simulink model "gm_sampleModel1869_3_sub_sub_sub"  (R2023a)
settings: Solver=VariableStepAuto  StartTime=0.0  StopTime=10.0  RelTol=1e-3
libraries: hdlsllib x3, simulink x3
settings Model: Creator=user1  LastModifiedBy=user1
settings OptimizationCC: BlockReduction=off  ConditionallyExecuteInputs=off
settings DebuggingCC: InheritedTsInSrcMsg=none

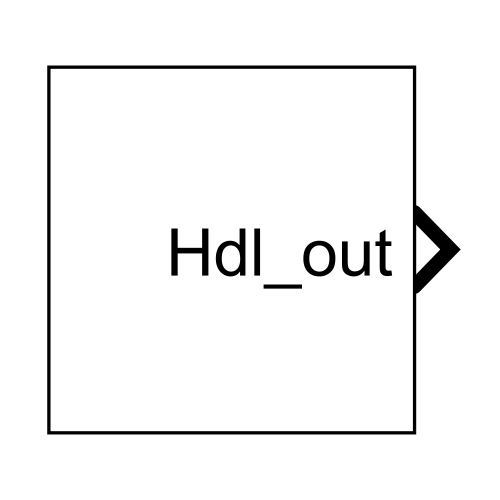
[thumbnail: Simulink's stored preview of the top-level diagram]
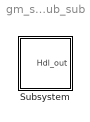
== system gm_sampleModel1869_3_sub_sub_sub ==
  Subsystem : Subsystem

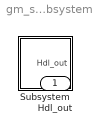
== system gm_sampleModel1869_3_sub_sub_sub/Subsystem ==
  Subsystem : Subsystem
  Hdl_out : Outport  OutDataTypeStr=uint8

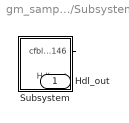
== system gm_sampleModel1869_3_sub_sub_sub/Subsystem/Subsystem ==
  Subsystem : Subsystem
  Hdl_out : Outport  OutDataTypeStr=uint8
  wires:
  Subsystem/1(cfblk146) -> Hdl_out/1

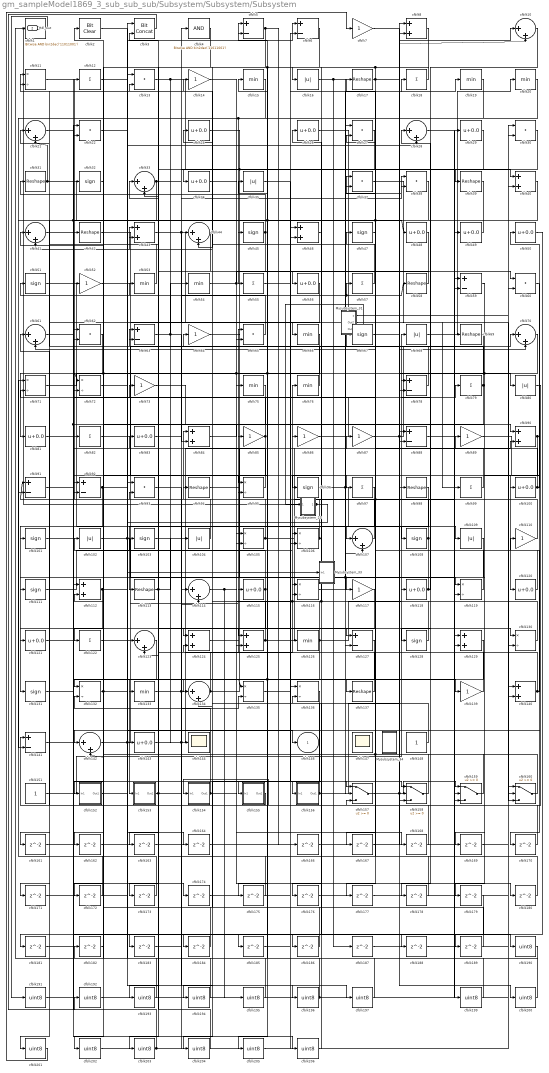
== system gm_sampleModel1869_3_sub_sub_sub/Subsystem/Subsystem/Subsystem ==
  Mysubsystem_23 : Subsystem  TreatAsAtomicUnit=on  RTWFcnName=Mysubsystem_23
      settings: RTWFcnNameOpts=User specified  RTWFileNameOpts=Use function name
  Mysubsystem_31 : Subsystem  TreatAsAtomicUnit=on  RTWFcnName=Mysubsystem_31
      settings: RTWFcnNameOpts=User specified  RTWFileNameOpts=Use function name
  Mysubsystem_33 : Subsystem  TreatAsAtomicUnit=on  RTWFcnName=Mysubsystem_33
      settings: RTWFcnNameOpts=User specified  RTWFileNameOpts=Use function name
  Mysubsystem_34 : Subsystem  TreatAsAtomicUnit=on  RTWFcnName=Mysubsystem_34
      settings: RTWFcnNameOpts=User specified  RTWFileNameOpts=Use function name
  cfblk1 : simulink/Logic and Bit Operations/Bitwise Operator  logicop=AND  UseBitMask=on  BitMask=bin2dec('11011001')  BitMaskRealWorld=Stored Integer
      settings: LibrarySourceBlock=|
      | hdlsllib/Logic and Bit
      | Operations/Bitwise
      | Operator
  cfblk{10,21,28,33,41,44,61,70,107,114,123,134,142} (13 alike) : Sum  Inputs=|++  OutDataTypeStr=uint8
  cfblk{24,26,29,34,48..50,56,81,83,100,115,118,120..121,143} (16 alike) : Bias  Bias=0.0  SaturateOnIntegerOverflow=off
  cfblk{32,45,47,51,67,96,101,103,108,111,128,131} (12 alike) : Signum
  cfblk{16,35,68,80,102,104,109} (7 alike) : Abs  OutDataTypeStr=uint8  SaturateOnIntegerOverflow=off
  cfblk{11,71..72,95,105..106,116,119,130,132,135..136} (12 alike) : Product  Inputs=*/  OutDataTypeStr=uint8  RndMeth=Zero  SaturateOnIntegerOverflow=on
  cfblk{7,14,52,64,73,85..87,89,110,117,139} (12 alike) : Gain  OutDataTypeStr=uint8
  cfblk{8,40,43,46,84,90,112,124..125,129,140} (11 alike) : Sum  OutDataTypeStr=uint8
  cfblk{17,31,39,42,58,69,94,98,113,137} (10 alike) : Reshape
  cfblk{12,18,55,57,79,82,97,99,122} (9 alike) : Sum  Inputs=+  OutDataTypeStr=uint8
  cfblk{15,19..20,53..54,66,75..76,126,133} (10 alike) : MinMax  OutDataTypeStr=uint8
  cfblk{5..6,59,63,78,88,91..92,127,141} (10 alike) : Sum  Inputs=+-  OutDataTypeStr=uint8
  cfblk{13,22,27,30,37..38,60,62,65,93} (10 alike) : DotProduct  OutDataTypeStr=uint8
  cfblk144 : Scope
  cfblk147 : Scope
      settings: Floating=on
  cfblk148 : Constant  OutDataTypeStr=uint8  SampleTime=-1
  cfblk151 : Constant  OutDataTypeStr=uint8  SampleTime=-1
  cfblk152 : Subsystem
      settings: LibrarySourceBlock=|
      | hdlsllib/Ports &
      | Subsystems/Subsystem
  cfblk153 : Subsystem
      settings: LibrarySourceBlock=|
      | hdlsllib/Ports &
      | Subsystems/Subsystem
  cfblk154 : Subsystem
      settings: LibrarySourceBlock=|
      | hdlsllib/Ports &
      | Subsystems/Subsystem
  cfblk155 : Subsystem
      settings: LibrarySourceBlock=|
      | hdlsllib/Ports &
      | Subsystems/Subsystem
  cfblk156 : Subsystem
      settings: LibrarySourceBlock=|
      | hdlsllib/Ports &
      | Subsystems/Subsystem
  cfblk{157..160} (4 alike) : Switch  OutDataTypeStr=uint8  SaturateOnIntegerOverflow=off  InputSameDT=off
  cfblk{161..164,166..189} (28 alike) : Delay  SampleTime=1
  cfblk{190..197,199..206} (16 alike) : DataTypeConversion  OutDataTypeStr=uint8  SaturateOnIntegerOverflow=off  RndMeth=Floor
  cfblk2 : simulink/Logic and Bit Operations/Bit Clear  iBit=0
      settings: LibrarySourceBlock=|
      | hdlsllib/Logic and Bit
      | Operations/Bit Clear
  cfblk3 : hdlsllib/Logic and Bit Operations/Bit Concat  numInputs=2
  cfblk4 : simulink/Logic and Bit Operations/Bitwise Operator  logicop=AND  UseBitMask=on  BitMask=bin2dec('11011001')  BitMaskRealWorld=Stored Integer
      settings: LibrarySourceBlock=|
      | hdlsllib/Logic and Bit
      | Operations/Bitwise
      | Operator
  cfblk146 : Outport  OutDataTypeStr=uint8  VectorParamsAs1DForOutWhenUnconnected=off
  Hdl_out : Outport  Port=2  OutDataTypeStr=uint8
  wires:
  Mysubsystem_31/3(Out3) -> Mysubsystem_23/1(In1)
  Mysubsystem_31/2(Out2) -> cfblk99/1
  Mysubsystem_31/1(y) -> cfblk40/2
  Mysubsystem_23/1(Out1) -> cfblk93/1, Hdl_out/1
  cfblk206/1 -> cfblk136/2
  cfblk141/1 -> cfblk206/1
  cfblk205/1 -> cfblk136/1
  cfblk129/1 -> cfblk205/1
  cfblk204/1 -> cfblk83/1
  cfblk136/1 -> cfblk204/1
  cfblk203/1 -> cfblk60/2, cfblk112/1
  cfblk202/1 -> cfblk4/1
  cfblk75/1 -> cfblk202/1
  cfblk201/1 -> cfblk7/1
  cfblk200/1 -> cfblk62/1
  cfblk7/1 -> cfblk200/1
  cfblk199/1 -> cfblk93/2
  cfblk88/1 -> cfblk199/1
  cfblk197/1 -> cfblk182/1
  cfblk93/1 -> cfblk197/1
  cfblk196/1 -> cfblk95/2, cfblk30/1
  cfblk195/1 -> cfblk2/1
  cfblk194/1 -> cfblk3/2
  cfblk179/1 -> cfblk194/1
  cfblk193/1 -> cfblk3/1
  cfblk27/1 -> cfblk193/1
  cfblk192/1 -> cfblk114/2
  cfblk3/1 -> cfblk192/1
  cfblk191/1 -> cfblk49/1
  cfblk1/1 -> cfblk191/1
  cfblk190/1 -> cfblk1/1
  cfblk161/1 -> cfblk190/1
  cfblk189/1 -> cfblk123/2
  cfblk188/1 -> cfblk159/3
  cfblk187/1 -> cfblk140/1
  cfblk186/1 -> cfblk124/2
  cfblk185/1 -> cfblk6/2
  cfblk184/1 -> cfblk112/2
  cfblk183/1 -> cfblk44/1
  cfblk48/1 -> cfblk183/1
  cfblk182/1 -> cfblk62/2
  cfblk181/1 -> cfblk22/1
  cfblk50/1 -> cfblk181/1
  cfblk180/1 -> cfblk27/2
  cfblk178/1 -> cfblk33/1
  cfblk10/1 -> cfblk178/1
  cfblk177/1 -> cfblk160/1
  cfblk29/1 -> cfblk177/1
  cfblk176/1 -> cfblk160/2
  cfblk97/1 -> cfblk176/1
  cfblk175/1 -> cfblk134/2
  cfblk174/1 -> cfblk46/2
  cfblk101/1 -> cfblk174/1
  cfblk173/1 -> cfblk71/1
  cfblk172/1 -> cfblk92/1
  cfblk32/1 -> cfblk172/1
  cfblk171/1 -> cfblk13/1
  cfblk56/1 -> cfblk171/1
  cfblk170/1 -> cfblk157/3
  cfblk169/1 -> cfblk30/2
  cfblk168/1 -> cfblk61/1
  cfblk167/1 -> cfblk59/2
  cfblk166/1 -> cfblk159/2
  cfblk164/1 -> cfblk8/1
  cfblk72/1 -> cfblk164/1
  cfblk163/1 -> cfblk114/1
  cfblk162/1 -> cfblk119/2
  cfblk61/1 -> cfblk124/1
  cfblk19/1 -> cfblk141/2
  cfblk76/1 -> cfblk11/1
  cfblk112/1 -> cfblk121/1, cfblk28/2
  cfblk65/1 -> cfblk51/1
  cfblk52/1 -> cfblk160/3
  cfblk6/1 -> cfblk44/2, cfblk95/1
  cfblk117/1 -> cfblk155/1(In1)
  cfblk44/1 -> cfblk143/1
  cfblk55/1 -> cfblk19/1
  cfblk102/1 -> cfblk123/1, cfblk129/2
  cfblk14/1 -> cfblk65/2
  cfblk79/1 -> cfblk5/1, cfblk162/1
  cfblk71/1 -> cfblk80/1
  cfblk66/1 -> cfblk135/1, cfblk175/1, cfblk101/1, cfblk125/2
  cfblk28/1 -> cfblk129/1
  cfblk64/1 -> cfblk70/1
  cfblk83/1 -> cfblk58/1, cfblk57/1
  cfblk81/1 -> cfblk134/1
  cfblk58/1 -> cfblk56/1
  cfblk20/1 -> cfblk33/2
  cfblk41/1 -> cfblk97/1
  cfblk133/1 -> cfblk126/1, cfblk38/2
  cfblk57/1 -> cfblk32/1
  cfblk69/1 -> cfblk128/1
  cfblk70/1 -> cfblk78/2, cfblk179/1
  cfblk11/1 -> cfblk48/1, cfblk130/2
  cfblk60/1 -> cfblk100/1
  cfblk49/1 -> cfblk45/1
  cfblk43/1 -> cfblk158/2, cfblk66/1
  cfblk5/1 -> cfblk142/2, cfblk72/1, cfblk166/1
  cfblk94/1 -> cfblk90/2
  cfblk22/1 -> cfblk106/2
  cfblk91/1 -> cfblk79/1
  cfblk63/1 -> cfblk84/2, cfblk54/1
  cfblk4/1 -> cfblk203/1
  cfblk35/1 -> cfblk158/1
  cfblk31/1 -> cfblk105/1, cfblk21/2
  cfblk159/1 -> cfblk37/2, cfblk41/1
  cfblk100/1 -> cfblk50/1, cfblk28/1
  cfblk135/1 -> cfblk87/1
  cfblk38/1 -> cfblk122/1
  cfblk53/1 -> cfblk21/1
  cfblk109/1 -> cfblk133/1
  cfblk111/1 -> cfblk106/1
  cfblk92/1 -> cfblk131/1, cfblk184/1
  cfblk153/1(Out1) -> cfblk73/1, cfblk189/1
  cfblk67/1 -> cfblk8/2
  cfblk78/1 -> cfblk43/1
  cfblk21/1 -> cfblk157/1, cfblk88/2
  cfblk39/1 -> cfblk91/2, cfblk167/1
  cfblk99/1 -> cfblk37/1
  cfblk115/1 -> cfblk72/2, cfblk163/1
  cfblk17/1 -> cfblk107/1, cfblk70/2
  cfblk131/1 -> cfblk22/2
  cfblk80/1 -> cfblk154/1(In1)
  cfblk86/1 -> cfblk59/1
  cfblk118/1 -> cfblk78/1, cfblk111/1
  cfblk96/1 -> cfblk108/1, cfblk158/3, cfblk38/1
  cfblk158/1 -> cfblk15/1
  cfblk73/1 -> cfblk127/2
  cfblk116/1 -> cfblk18/1
  cfblk152/1(Out1) -> cfblk6/1
  cfblk137/1 -> cfblk14/1
  cfblk142/1 -> Mysubsystem_33/1(In1), cfblk115/1
  cfblk59/1 -> cfblk119/1
  cfblk12/1 -> cfblk139/1
  cfblk113/1 -> cfblk13/2, cfblk104/1
  cfblk13/1 -> cfblk40/1, cfblk144/1
  cfblk123/1 -> cfblk153/1(In1)
  cfblk84/1 -> cfblk90/1
  cfblk108/1 -> cfblk157/2, cfblk161/1, cfblk5/2
  cfblk120/1 -> cfblk91/1, cfblk71/2
  cfblk37/1 -> cfblk140/2
  cfblk18/1 -> cfblk16/1
  cfblk85/1 -> cfblk132/1, cfblk53/1
  cfblk104/1 -> cfblk63/1
  cfblk105/1 -> cfblk69/1, cfblk24/1
  cfblk90/1 -> cfblk169/1, cfblk170/1
  cfblk42/1 -> cfblk120/1
  cfblk132/1 -> cfblk52/1, cfblk146/1
  cfblk121/1 -> cfblk82/1
  cfblk134/1 -> cfblk46/1, cfblk103/1
  cfblk47/1 -> cfblk17/1
  cfblk16/1 -> cfblk130/1, cfblk187/1
  cfblk119/1 -> cfblk61/2
  cfblk54/1 -> cfblk60/1, cfblk180/1
  cfblk46/1 -> cfblk96/1
  cfblk154/1(Out1) -> cfblk132/2, cfblk168/1
  cfblk160/1 -> cfblk47/1, cfblk63/2
  cfblk106/1 -> cfblk42/1, cfblk156/1(In1)
  cfblk148/1 -> cfblk102/1
  cfblk127/1 -> cfblk152/1(In1)
  cfblk130/1 -> cfblk35/1
  cfblk34/1 -> cfblk75/1
  cfblk157/1 -> cfblk159/1, cfblk10/1
  cfblk124/1 -> cfblk127/1
  cfblk156/1(Out1) -> cfblk88/1, cfblk11/2
  cfblk2/1 -> cfblk196/1
  cfblk15/1 -> cfblk55/1, cfblk173/1
  cfblk45/1 -> cfblk31/1, cfblk105/2
  cfblk26/1 -> cfblk98/1
  cfblk125/1 -> cfblk89/1, cfblk41/2
  cfblk95/1 -> cfblk12/1
  cfblk62/1 -> cfblk81/1
  cfblk87/1 -> cfblk29/1, cfblk10/2
  cfblk51/1 -> cfblk109/1
  cfblk33/1 -> cfblk39/1, cfblk92/2
  cfblk98/1 -> cfblk113/1
  cfblk122/1 -> cfblk64/1
  cfblk128/1 -> cfblk94/1, cfblk116/1, cfblk26/1
  cfblk40/1 -> cfblk125/1, cfblk201/1
  cfblk143/1 -> cfblk27/1, cfblk135/2, cfblk188/1
  cfblk155/1(Out1) -> cfblk141/1
  cfblk151/1 -> cfblk118/1
  cfblk126/1 -> cfblk68/1, cfblk43/2, cfblk185/1
  cfblk103/1 -> cfblk85/1
  cfblk107/1 -> cfblk84/1
  cfblk139/1 -> cfblk65/1
  cfblk24/1 -> cfblk117/1, cfblk107/2
  cfblk89/1 -> cfblk142/1
  cfblk8/1 -> cfblk137/1, cfblk186/1
  cfblk30/1 -> cfblk34/1
  cfblk140/1 -> cfblk86/1, cfblk110/1
  cfblk114/1 -> cfblk116/2, cfblk195/1
  cfblk68/1 -> cfblk20/1
  cfblk82/1 -> cfblk67/1
  cfblk110/1 -> cfblk76/1

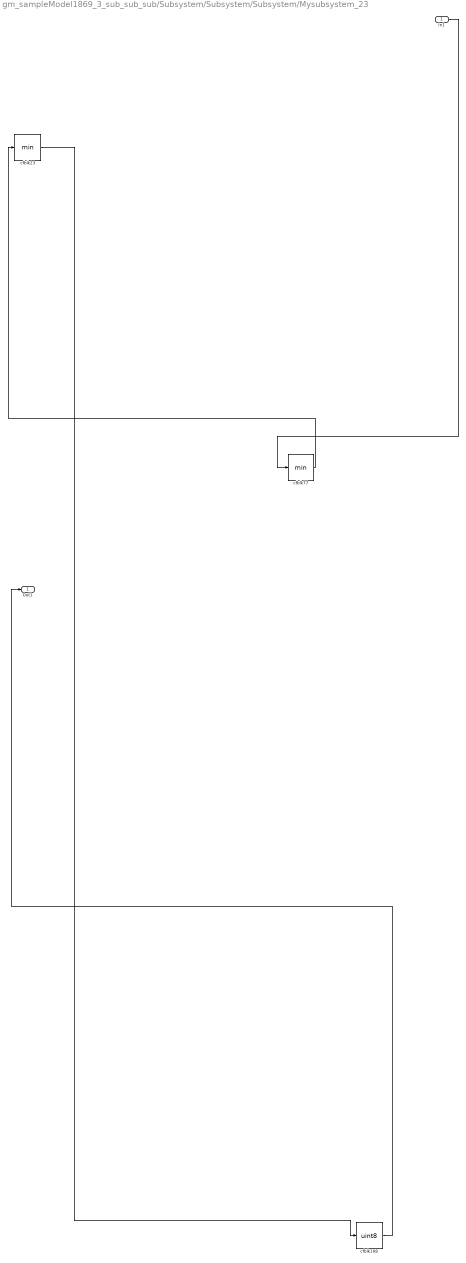
== system gm_sampleModel1869_3_sub_sub_sub/Subsystem/Subsystem/Subsystem/Mysubsystem_23 ==
  In1 : Inport
  cfblk198 : DataTypeConversion  OutDataTypeStr=uint8  SaturateOnIntegerOverflow=off  RndMeth=Floor
  cfblk23 : MinMax
  cfblk77 : MinMax
  Out1 : Outport
  wires:
  cfblk198/1 -> Out1/1
  cfblk77/1 -> cfblk23/1
  In1/1 -> cfblk77/1
  cfblk23/1 -> cfblk198/1

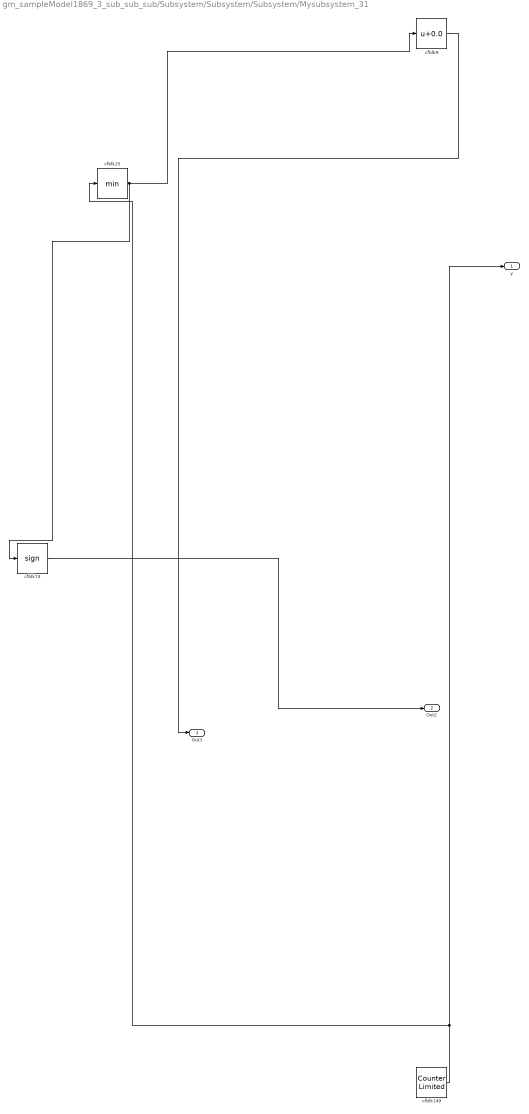
== system gm_sampleModel1869_3_sub_sub_sub/Subsystem/Subsystem/Subsystem/Mysubsystem_31 ==
  cfblk149 : hdlsllib/Sources/Counter Limited  uplimit=7  tsamp=-1
  cfblk25 : MinMax
  cfblk74 : Signum
  cfblk9 : Bias  Bias=0.0  SaturateOnIntegerOverflow=off
  y : Outport
  Out2 : Outport  Port=2
  Out3 : Outport  Port=3
  wires:
  cfblk149/1 -> y/1, cfblk25/1
  cfblk25/1 -> cfblk74/1, cfblk9/1
  cfblk74/1 -> Out2/1
  cfblk9/1 -> Out3/1

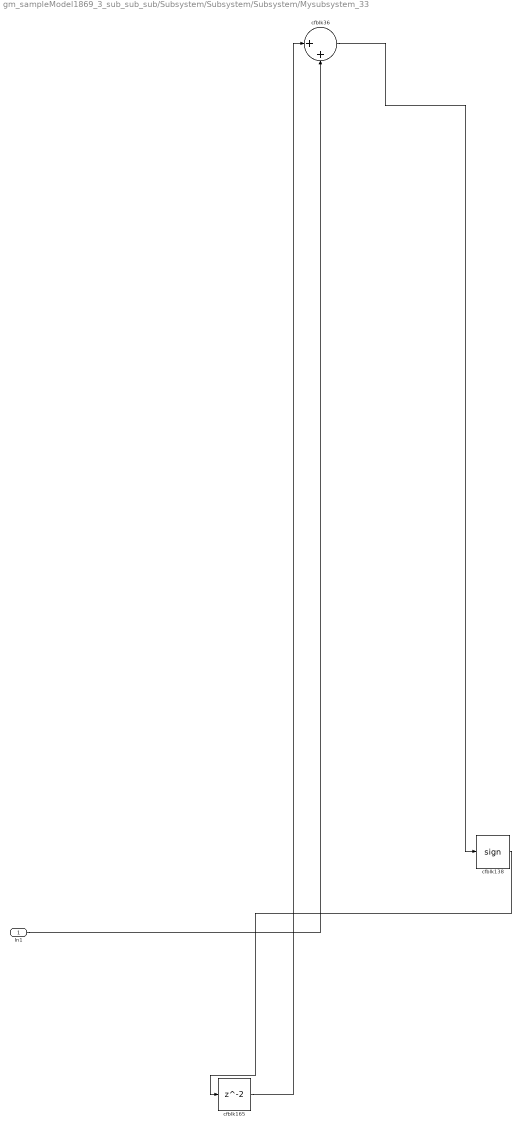
== system gm_sampleModel1869_3_sub_sub_sub/Subsystem/Subsystem/Subsystem/Mysubsystem_33 ==
  In1 : Inport
  cfblk138 : Signum
  cfblk165 : Delay  SampleTime=1
  cfblk36 : Sum  Inputs=|++
  wires:
  In1/1 -> cfblk36/2
  cfblk36/1 -> cfblk138/1
  cfblk165/1 -> cfblk36/1
  cfblk138/1 -> cfblk165/1

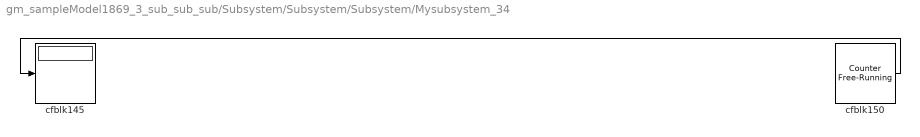
== system gm_sampleModel1869_3_sub_sub_sub/Subsystem/Subsystem/Subsystem/Mysubsystem_34 ==
  cfblk145 : Display
  cfblk150 : hdlsllib/Sources/Counter Free-Running  NumBits=16  tsamp=-1
  wires:
  cfblk150/1 -> cfblk145/1

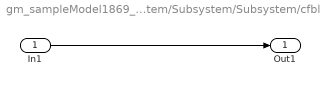
== system gm_sampleModel1869_3_sub_sub_sub/Subsystem/Subsystem/Subsystem/cfblk152 ==
  In1 : Inport
  Out1 : Outport
  wires:
  In1/1 -> Out1/1

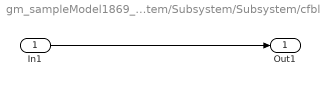
== system gm_sampleModel1869_3_sub_sub_sub/Subsystem/Subsystem/Subsystem/cfblk153 ==
  In1 : Inport
  Out1 : Outport
  wires:
  In1/1 -> Out1/1

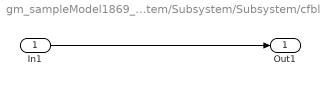
== system gm_sampleModel1869_3_sub_sub_sub/Subsystem/Subsystem/Subsystem/cfblk154 ==
  In1 : Inport
  Out1 : Outport
  wires:
  In1/1 -> Out1/1

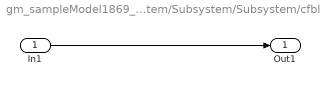
== system gm_sampleModel1869_3_sub_sub_sub/Subsystem/Subsystem/Subsystem/cfblk155 ==
  In1 : Inport
  Out1 : Outport
  wires:
  In1/1 -> Out1/1

== system gm_sampleModel1869_3_sub_sub_sub/Subsystem/Subsystem/Subsystem/cfblk156 ==
  In1 : Inport
  Out1 : Outport
  wires:
  In1/1 -> Out1/1
